simulink model "Assem4"  (R2018b)
(part 2 of 15)

  Revolute50 : sm_lib/Joints/Revolute Joint  SenseConstraintForce=off  SenseConstraintForceX=off  SenseConstraintForceY=off  SenseConstraintForceZ=off  SenseConstraintTorque=off  SenseConstraintTorqueX=off  SenseConstraintTorqueY=off  SenseConstraintTorqueZ=off  SenseTotalForce=off  SenseTotalForceX=off  SenseTotalForceY=off  SenseTotalForceZ=off  SenseTotalTorque=off  SenseTotalTorqueX=off  SenseTotalTorqueY=off  SenseTotalTorqueZ=off  CompositeWrenchDir=FollowerOnBase  CompositeWrenchFrame=BaseFrame  EquilibriumPosition=0  EquilibriumPositionUnits=rad  SpringStiffness=0  SpringStiffnessUnits=N*m/rad  DampingCoefficient=0  DampingCoefficientUnits=N*m/(rad/s)  TorqueActuationMode=NoTorque  MotionActuationMode=ComputedMotion  SensePosition=off  SenseVelocity=off  SenseAcceleration=off  SenseTorqueForce=off  PositionTargetSpecify=on  PositionTargetPriority=Low  PositionTargetValue=smiData.RevoluteJoint(51).Rz.Pos  PositionTargetValueUnits=deg  VelocityTargetSpecify=off  VelocityTargetPriority=High  VelocityTargetValue=0  VelocityTargetValueUnits=deg/s
  Revolute51 : sm_lib/Joints/Revolute Joint  SenseConstraintForce=off  SenseConstraintForceX=off  SenseConstraintForceY=off  SenseConstraintForceZ=off  SenseConstraintTorque=off  SenseConstraintTorqueX=off  SenseConstraintTorqueY=off  SenseConstraintTorqueZ=off  SenseTotalForce=off  SenseTotalForceX=off  SenseTotalForceY=off  SenseTotalForceZ=off  SenseTotalTorque=off  SenseTotalTorqueX=off  SenseTotalTorqueY=off  SenseTotalTorqueZ=off  CompositeWrenchDir=FollowerOnBase  CompositeWrenchFrame=BaseFrame  EquilibriumPosition=0  EquilibriumPositionUnits=rad  SpringStiffness=0  SpringStiffnessUnits=N*m/rad  DampingCoefficient=0  DampingCoefficientUnits=N*m/(rad/s)  TorqueActuationMode=NoTorque  MotionActuationMode=ComputedMotion  SensePosition=off  SenseVelocity=off  SenseAcceleration=off  SenseTorqueForce=off  PositionTargetSpecify=on  PositionTargetPriority=Low  PositionTargetValue=smiData.RevoluteJoint(52).Rz.Pos  PositionTargetValueUnits=deg  VelocityTargetSpecify=off  VelocityTargetPriority=High  VelocityTargetValue=0  VelocityTargetValueUnits=deg/s
  Revolute52 : sm_lib/Joints/Revolute Joint  SenseConstraintForce=off  SenseConstraintForceX=off  SenseConstraintForceY=off  SenseConstraintForceZ=off  SenseConstraintTorque=off  SenseConstraintTorqueX=off  SenseConstraintTorqueY=off  SenseConstraintTorqueZ=off  SenseTotalForce=off  SenseTotalForceX=off  SenseTotalForceY=off  SenseTotalForceZ=off  SenseTotalTorque=off  SenseTotalTorqueX=off  SenseTotalTorqueY=off  SenseTotalTorqueZ=off  CompositeWrenchDir=FollowerOnBase  CompositeWrenchFrame=BaseFrame  EquilibriumPosition=0  EquilibriumPositionUnits=rad  SpringStiffness=0  SpringStiffnessUnits=N*m/rad  DampingCoefficient=0  DampingCoefficientUnits=N*m/(rad/s)  TorqueActuationMode=NoTorque  MotionActuationMode=ComputedMotion  SensePosition=off  SenseVelocity=off  SenseAcceleration=off  SenseTorqueForce=off  PositionTargetSpecify=on  PositionTargetPriority=Low  PositionTargetValue=smiData.RevoluteJoint(53).Rz.Pos  PositionTargetValueUnits=deg  VelocityTargetSpecify=off  VelocityTargetPriority=High  VelocityTargetValue=0  VelocityTargetValueUnits=deg/s
  Revolute53 : sm_lib/Joints/Revolute Joint  SenseConstraintForce=off  SenseConstraintForceX=off  SenseConstraintForceY=off  SenseConstraintForceZ=off  SenseConstraintTorque=off  SenseConstraintTorqueX=off  SenseConstraintTorqueY=off  SenseConstraintTorqueZ=off  SenseTotalForce=off  SenseTotalForceX=off  SenseTotalForceY=off  SenseTotalForceZ=off  SenseTotalTorque=off  SenseTotalTorqueX=off  SenseTotalTorqueY=off  SenseTotalTorqueZ=off  CompositeWrenchDir=FollowerOnBase  CompositeWrenchFrame=BaseFrame  EquilibriumPosition=0  EquilibriumPositionUnits=rad  SpringStiffness=0  SpringStiffnessUnits=N*m/rad  DampingCoefficient=0  DampingCoefficientUnits=N*m/(rad/s)  TorqueActuationMode=NoTorque  MotionActuationMode=ComputedMotion  SensePosition=off  SenseVelocity=off  SenseAcceleration=off  SenseTorqueForce=off  PositionTargetSpecify=on  PositionTargetPriority=Low  PositionTargetValue=smiData.RevoluteJoint(54).Rz.Pos  PositionTargetValueUnits=deg  VelocityTargetSpecify=off  VelocityTargetPriority=High  VelocityTargetValue=0  VelocityTargetValueUnits=deg/s
  Revolute54 : sm_lib/Joints/Revolute Joint  SenseConstraintForce=off  SenseConstraintForceX=off  SenseConstraintForceY=off  SenseConstraintForceZ=off  SenseConstraintTorque=off  SenseConstraintTorqueX=off  SenseConstraintTorqueY=off  SenseConstraintTorqueZ=off  SenseTotalForce=off  SenseTotalForceX=off  SenseTotalForceY=off  SenseTotalForceZ=off  SenseTotalTorque=off  SenseTotalTorqueX=off  SenseTotalTorqueY=off  SenseTotalTorqueZ=off  CompositeWrenchDir=FollowerOnBase  CompositeWrenchFrame=BaseFrame  EquilibriumPosition=0  EquilibriumPositionUnits=rad  SpringStiffness=0  SpringStiffnessUnits=N*m/rad  DampingCoefficient=0  DampingCoefficientUnits=N*m/(rad/s)  TorqueActuationMode=NoTorque  MotionActuationMode=ComputedMotion  SensePosition=off  SenseVelocity=off  SenseAcceleration=off  SenseTorqueForce=off  PositionTargetSpecify=on  PositionTargetPriority=Low  PositionTargetValue=smiData.RevoluteJoint(55).Rz.Pos  PositionTargetValueUnits=deg  VelocityTargetSpecify=off  VelocityTargetPriority=High  VelocityTargetValue=0  VelocityTargetValueUnits=deg/s
  Revolute55 : sm_lib/Joints/Revolute Joint  SenseConstraintForce=off  SenseConstraintForceX=off  SenseConstraintForceY=off  SenseConstraintForceZ=off  SenseConstraintTorque=off  SenseConstraintTorqueX=off  SenseConstraintTorqueY=off  SenseConstraintTorqueZ=off  SenseTotalForce=off  SenseTotalForceX=off  SenseTotalForceY=off  SenseTotalForceZ=off  SenseTotalTorque=off  SenseTotalTorqueX=off  SenseTotalTorqueY=off  SenseTotalTorqueZ=off  CompositeWrenchDir=FollowerOnBase  CompositeWrenchFrame=BaseFrame  EquilibriumPosition=0  EquilibriumPositionUnits=rad  SpringStiffness=0  SpringStiffnessUnits=N*m/rad  DampingCoefficient=0  DampingCoefficientUnits=N*m/(rad/s)  TorqueActuationMode=NoTorque  MotionActuationMode=ComputedMotion  SensePosition=off  SenseVelocity=off  SenseAcceleration=off  SenseTorqueForce=off  PositionTargetSpecify=on  PositionTargetPriority=Low  PositionTargetValue=smiData.RevoluteJoint(56).Rz.Pos  PositionTargetValueUnits=deg  VelocityTargetSpecify=off  VelocityTargetPriority=High  VelocityTargetValue=0  VelocityTargetValueUnits=deg/s
  Revolute56 : sm_lib/Joints/Revolute Joint  SenseConstraintForce=off  SenseConstraintForceX=off  SenseConstraintForceY=off  SenseConstraintForceZ=off  SenseConstraintTorque=off  SenseConstraintTorqueX=off  SenseConstraintTorqueY=off  SenseConstraintTorqueZ=off  SenseTotalForce=off  SenseTotalForceX=off  SenseTotalForceY=off  SenseTotalForceZ=off  SenseTotalTorque=off  SenseTotalTorqueX=off  SenseTotalTorqueY=off  SenseTotalTorqueZ=off  CompositeWrenchDir=FollowerOnBase  CompositeWrenchFrame=BaseFrame  EquilibriumPosition=0  EquilibriumPositionUnits=rad  SpringStiffness=0  SpringStiffnessUnits=N*m/rad  DampingCoefficient=0  DampingCoefficientUnits=N*m/(rad/s)  TorqueActuationMode=NoTorque  MotionActuationMode=ComputedMotion  SensePosition=off  SenseVelocity=off  SenseAcceleration=off  SenseTorqueForce=off  PositionTargetSpecify=on  PositionTargetPriority=Low  PositionTargetValue=smiData.RevoluteJoint(57).Rz.Pos  PositionTargetValueUnits=deg  VelocityTargetSpecify=off  VelocityTargetPriority=High  VelocityTargetValue=0  VelocityTargetValueUnits=deg/s
  Revolute57 : sm_lib/Joints/Revolute Joint  SenseConstraintForce=off  SenseConstraintForceX=off  SenseConstraintForceY=off  SenseConstraintForceZ=off  SenseConstraintTorque=off  SenseConstraintTorqueX=off  SenseConstraintTorqueY=off  SenseConstraintTorqueZ=off  SenseTotalForce=off  SenseTotalForceX=off  SenseTotalForceY=off  SenseTotalForceZ=off  SenseTotalTorque=off  SenseTotalTorqueX=off  SenseTotalTorqueY=off  SenseTotalTorqueZ=off  CompositeWrenchDir=FollowerOnBase  CompositeWrenchFrame=BaseFrame  EquilibriumPosition=0  EquilibriumPositionUnits=rad  SpringStiffness=0  SpringStiffnessUnits=N*m/rad  DampingCoefficient=0  DampingCoefficientUnits=N*m/(rad/s)  TorqueActuationMode=NoTorque  MotionActuationMode=ComputedMotion  SensePosition=off  SenseVelocity=off  SenseAcceleration=off  SenseTorqueForce=off  PositionTargetSpecify=on  PositionTargetPriority=Low  PositionTargetValue=smiData.RevoluteJoint(58).Rz.Pos  PositionTargetValueUnits=deg  VelocityTargetSpecify=off  VelocityTargetPriority=High  VelocityTargetValue=0  VelocityTargetValueUnits=deg/s
  Revolute58 : sm_lib/Joints/Revolute Joint  SenseConstraintForce=off  SenseConstraintForceX=off  SenseConstraintForceY=off  SenseConstraintForceZ=off  SenseConstraintTorque=off  SenseConstraintTorqueX=off  SenseConstraintTorqueY=off  SenseConstraintTorqueZ=off  SenseTotalForce=off  SenseTotalForceX=off  SenseTotalForceY=off  SenseTotalForceZ=off  SenseTotalTorque=off  SenseTotalTorqueX=off  SenseTotalTorqueY=off  SenseTotalTorqueZ=off  CompositeWrenchDir=FollowerOnBase  CompositeWrenchFrame=BaseFrame  EquilibriumPosition=0  EquilibriumPositionUnits=rad  SpringStiffness=0  SpringStiffnessUnits=N*m/rad  DampingCoefficient=0  DampingCoefficientUnits=N*m/(rad/s)  TorqueActuationMode=NoTorque  MotionActuationMode=ComputedMotion  SensePosition=off  SenseVelocity=off  SenseAcceleration=off  SenseTorqueForce=off  PositionTargetSpecify=on  PositionTargetPriority=Low  PositionTargetValue=smiData.RevoluteJoint(59).Rz.Pos  PositionTargetValueUnits=deg  VelocityTargetSpecify=off  VelocityTargetPriority=High  VelocityTargetValue=0  VelocityTargetValueUnits=deg/s
  Revolute59 : sm_lib/Joints/Revolute Joint  SenseConstraintForce=off  SenseConstraintForceX=off  SenseConstraintForceY=off  SenseConstraintForceZ=off  SenseConstraintTorque=off  SenseConstraintTorqueX=off  SenseConstraintTorqueY=off  SenseConstraintTorqueZ=off  SenseTotalForce=off  SenseTotalForceX=off  SenseTotalForceY=off  SenseTotalForceZ=off  SenseTotalTorque=off  SenseTotalTorqueX=off  SenseTotalTorqueY=off  SenseTotalTorqueZ=off  CompositeWrenchDir=FollowerOnBase  CompositeWrenchFrame=BaseFrame  EquilibriumPosition=0  EquilibriumPositionUnits=rad  SpringStiffness=0  SpringStiffnessUnits=N*m/rad  DampingCoefficient=0  DampingCoefficientUnits=N*m/(rad/s)  TorqueActuationMode=NoTorque  MotionActuationMode=ComputedMotion  SensePosition=off  SenseVelocity=off  SenseAcceleration=off  SenseTorqueForce=off  PositionTargetSpecify=on  PositionTargetPriority=Low  PositionTargetValue=smiData.RevoluteJoint(60).Rz.Pos  PositionTargetValueUnits=deg  VelocityTargetSpecify=off  VelocityTargetPriority=High  VelocityTargetValue=0  VelocityTargetValueUnits=deg/s
  Revolute6 : sm_lib/Joints/Revolute Joint  SenseConstraintForce=off  SenseConstraintForceX=off  SenseConstraintForceY=off  SenseConstraintForceZ=off  SenseConstraintTorque=off  SenseConstraintTorqueX=off  SenseConstraintTorqueY=off  SenseConstraintTorqueZ=off  SenseTotalForce=off  SenseTotalForceX=off  SenseTotalForceY=off  SenseTotalForceZ=off  SenseTotalTorque=off  SenseTotalTorqueX=off  SenseTotalTorqueY=off  SenseTotalTorqueZ=off  CompositeWrenchDir=FollowerOnBase  CompositeWrenchFrame=BaseFrame  EquilibriumPosition=0  EquilibriumPositionUnits=rad  SpringStiffness=0  SpringStiffnessUnits=N*m/rad  DampingCoefficient=0  DampingCoefficientUnits=N*m/(rad/s)  TorqueActuationMode=NoTorque  MotionActuationMode=ComputedMotion  SensePosition=off  SenseVelocity=off  SenseAcceleration=off  SenseTorqueForce=off  PositionTargetSpecify=on  PositionTargetPriority=Low  PositionTargetValue=smiData.RevoluteJoint(7).Rz.Pos  PositionTargetValueUnits=deg  VelocityTargetSpecify=off  VelocityTargetPriority=High  VelocityTargetValue=0  VelocityTargetValueUnits=deg/s
  Revolute60 : sm_lib/Joints/Revolute Joint  SenseConstraintForce=off  SenseConstraintForceX=off  SenseConstraintForceY=off  SenseConstraintForceZ=off  SenseConstraintTorque=off  SenseConstraintTorqueX=off  SenseConstraintTorqueY=off  SenseConstraintTorqueZ=off  SenseTotalForce=off  SenseTotalForceX=off  SenseTotalForceY=off  SenseTotalForceZ=off  SenseTotalTorque=off  SenseTotalTorqueX=off  SenseTotalTorqueY=off  SenseTotalTorqueZ=off  CompositeWrenchDir=FollowerOnBase  CompositeWrenchFrame=BaseFrame  EquilibriumPosition=0  EquilibriumPositionUnits=rad  SpringStiffness=0  SpringStiffnessUnits=N*m/rad  DampingCoefficient=0  DampingCoefficientUnits=N*m/(rad/s)  TorqueActuationMode=NoTorque  MotionActuationMode=ComputedMotion  SensePosition=off  SenseVelocity=off  SenseAcceleration=off  SenseTorqueForce=off  PositionTargetSpecify=on  PositionTargetPriority=Low  PositionTargetValue=smiData.RevoluteJoint(61).Rz.Pos  PositionTargetValueUnits=deg  VelocityTargetSpecify=off  VelocityTargetPriority=High  VelocityTargetValue=0  VelocityTargetValueUnits=deg/s
  Revolute61 : sm_lib/Joints/Revolute Joint  SenseConstraintForce=off  SenseConstraintForceX=off  SenseConstraintForceY=off  SenseConstraintForceZ=off  SenseConstraintTorque=off  SenseConstraintTorqueX=off  SenseConstraintTorqueY=off  SenseConstraintTorqueZ=off  SenseTotalForce=off  SenseTotalForceX=off  SenseTotalForceY=off  SenseTotalForceZ=off  SenseTotalTorque=off  SenseTotalTorqueX=off  SenseTotalTorqueY=off  SenseTotalTorqueZ=off  CompositeWrenchDir=FollowerOnBase  CompositeWrenchFrame=BaseFrame  EquilibriumPosition=0  EquilibriumPositionUnits=rad  SpringStiffness=0  SpringStiffnessUnits=N*m/rad  DampingCoefficient=0  DampingCoefficientUnits=N*m/(rad/s)  TorqueActuationMode=NoTorque  MotionActuationMode=ComputedMotion  SensePosition=off  SenseVelocity=off  SenseAcceleration=off  SenseTorqueForce=off  PositionTargetSpecify=on  PositionTargetPriority=Low  PositionTargetValue=smiData.RevoluteJoint(62).Rz.Pos  PositionTargetValueUnits=deg  VelocityTargetSpecify=off  VelocityTargetPriority=High  VelocityTargetValue=0  VelocityTargetValueUnits=deg/s
  Revolute62 : sm_lib/Joints/Revolute Joint  SenseConstraintForce=off  SenseConstraintForceX=off  SenseConstraintForceY=off  SenseConstraintForceZ=off  SenseConstraintTorque=off  SenseConstraintTorqueX=off  SenseConstraintTorqueY=off  SenseConstraintTorqueZ=off  SenseTotalForce=off  SenseTotalForceX=off  SenseTotalForceY=off  SenseTotalForceZ=off  SenseTotalTorque=off  SenseTotalTorqueX=off  SenseTotalTorqueY=off  SenseTotalTorqueZ=off  CompositeWrenchDir=FollowerOnBase  CompositeWrenchFrame=BaseFrame  EquilibriumPosition=0  EquilibriumPositionUnits=rad  SpringStiffness=0  SpringStiffnessUnits=N*m/rad  DampingCoefficient=0  DampingCoefficientUnits=N*m/(rad/s)  TorqueActuationMode=NoTorque  MotionActuationMode=ComputedMotion  SensePosition=off  SenseVelocity=off  SenseAcceleration=off  SenseTorqueForce=off  PositionTargetSpecify=on  PositionTargetPriority=Low  PositionTargetValue=smiData.RevoluteJoint(63).Rz.Pos  PositionTargetValueUnits=deg  VelocityTargetSpecify=off  VelocityTargetPriority=High  VelocityTargetValue=0  VelocityTargetValueUnits=deg/s
  Revolute63 : sm_lib/Joints/Revolute Joint  SenseConstraintForce=off  SenseConstraintForceX=off  SenseConstraintForceY=off  SenseConstraintForceZ=off  SenseConstraintTorque=off  SenseConstraintTorqueX=off  SenseConstraintTorqueY=off  SenseConstraintTorqueZ=off  SenseTotalForce=off  SenseTotalForceX=off  SenseTotalForceY=off  SenseTotalForceZ=off  SenseTotalTorque=off  SenseTotalTorqueX=off  SenseTotalTorqueY=off  SenseTotalTorqueZ=off  CompositeWrenchDir=FollowerOnBase  CompositeWrenchFrame=BaseFrame  EquilibriumPosition=0  EquilibriumPositionUnits=rad  SpringStiffness=0  SpringStiffnessUnits=N*m/rad  DampingCoefficient=0  DampingCoefficientUnits=N*m/(rad/s)  TorqueActuationMode=NoTorque  MotionActuationMode=ComputedMotion  SensePosition=off  SenseVelocity=off  SenseAcceleration=off  SenseTorqueForce=off  PositionTargetSpecify=on  PositionTargetPriority=Low  PositionTargetValue=smiData.RevoluteJoint(64).Rz.Pos  PositionTargetValueUnits=deg  VelocityTargetSpecify=off  VelocityTargetPriority=High  VelocityTargetValue=0  VelocityTargetValueUnits=deg/s
  Revolute64 : sm_lib/Joints/Revolute Joint  SenseConstraintForce=off  SenseConstraintForceX=off  SenseConstraintForceY=off  SenseConstraintForceZ=off  SenseConstraintTorque=off  SenseConstraintTorqueX=off  SenseConstraintTorqueY=off  SenseConstraintTorqueZ=off  SenseTotalForce=off  SenseTotalForceX=off  SenseTotalForceY=off  SenseTotalForceZ=off  SenseTotalTorque=off  SenseTotalTorqueX=off  SenseTotalTorqueY=off  SenseTotalTorqueZ=off  CompositeWrenchDir=FollowerOnBase  CompositeWrenchFrame=BaseFrame  EquilibriumPosition=0  EquilibriumPositionUnits=rad  SpringStiffness=0  SpringStiffnessUnits=N*m/rad  DampingCoefficient=0  DampingCoefficientUnits=N*m/(rad/s)  TorqueActuationMode=NoTorque  MotionActuationMode=ComputedMotion  SensePosition=off  SenseVelocity=off  SenseAcceleration=off  SenseTorqueForce=off  PositionTargetSpecify=on  PositionTargetPriority=Low  PositionTargetValue=smiData.RevoluteJoint(65).Rz.Pos  PositionTargetValueUnits=deg  VelocityTargetSpecify=off  VelocityTargetPriority=High  VelocityTargetValue=0  VelocityTargetValueUnits=deg/s
  Revolute65 : sm_lib/Joints/Revolute Joint  SenseConstraintForce=off  SenseConstraintForceX=off  SenseConstraintForceY=off  SenseConstraintForceZ=off  SenseConstraintTorque=off  SenseConstraintTorqueX=off  SenseConstraintTorqueY=off  SenseConstraintTorqueZ=off  SenseTotalForce=off  SenseTotalForceX=off  SenseTotalForceY=off  SenseTotalForceZ=off  SenseTotalTorque=off  SenseTotalTorqueX=off  SenseTotalTorqueY=off  SenseTotalTorqueZ=off  CompositeWrenchDir=FollowerOnBase  CompositeWrenchFrame=BaseFrame  EquilibriumPosition=0  EquilibriumPositionUnits=rad  SpringStiffness=0  SpringStiffnessUnits=N*m/rad  DampingCoefficient=0  DampingCoefficientUnits=N*m/(rad/s)  TorqueActuationMode=NoTorque  MotionActuationMode=ComputedMotion  SensePosition=off  SenseVelocity=off  SenseAcceleration=off  SenseTorqueForce=off  PositionTargetSpecify=on  PositionTargetPriority=Low  PositionTargetValue=smiData.RevoluteJoint(66).Rz.Pos  PositionTargetValueUnits=deg  VelocityTargetSpecify=off  VelocityTargetPriority=High  VelocityTargetValue=0  VelocityTargetValueUnits=deg/s
  Revolute66 : sm_lib/Joints/Revolute Joint  SenseConstraintForce=off  SenseConstraintForceX=off  SenseConstraintForceY=off  SenseConstraintForceZ=off  SenseConstraintTorque=off  SenseConstraintTorqueX=off  SenseConstraintTorqueY=off  SenseConstraintTorqueZ=off  SenseTotalForce=off  SenseTotalForceX=off  SenseTotalForceY=off  SenseTotalForceZ=off  SenseTotalTorque=off  SenseTotalTorqueX=off  SenseTotalTorqueY=off  SenseTotalTorqueZ=off  CompositeWrenchDir=FollowerOnBase  CompositeWrenchFrame=BaseFrame  EquilibriumPosition=0  EquilibriumPositionUnits=rad  SpringStiffness=0  SpringStiffnessUnits=N*m/rad  DampingCoefficient=0  DampingCoefficientUnits=N*m/(rad/s)  TorqueActuationMode=NoTorque  MotionActuationMode=ComputedMotion  SensePosition=off  SenseVelocity=off  SenseAcceleration=off  SenseTorqueForce=off  PositionTargetSpecify=on  PositionTargetPriority=Low  PositionTargetValue=smiData.RevoluteJoint(67).Rz.Pos  PositionTargetValueUnits=deg  VelocityTargetSpecify=off  VelocityTargetPriority=High  VelocityTargetValue=0  VelocityTargetValueUnits=deg/s
  Revolute67 : sm_lib/Joints/Revolute Joint  SenseConstraintForce=off  SenseConstraintForceX=off  SenseConstraintForceY=off  SenseConstraintForceZ=off  SenseConstraintTorque=off  SenseConstraintTorqueX=off  SenseConstraintTorqueY=off  SenseConstraintTorqueZ=off  SenseTotalForce=off  SenseTotalForceX=off  SenseTotalForceY=off  SenseTotalForceZ=off  SenseTotalTorque=off  SenseTotalTorqueX=off  SenseTotalTorqueY=off  SenseTotalTorqueZ=off  CompositeWrenchDir=FollowerOnBase  CompositeWrenchFrame=BaseFrame  EquilibriumPosition=0  EquilibriumPositionUnits=rad  SpringStiffness=0  SpringStiffnessUnits=N*m/rad  DampingCoefficient=0  DampingCoefficientUnits=N*m/(rad/s)  TorqueActuationMode=NoTorque  MotionActuationMode=ComputedMotion  SensePosition=off  SenseVelocity=off  SenseAcceleration=off  SenseTorqueForce=off  PositionTargetSpecify=on  PositionTargetPriority=Low  PositionTargetValue=smiData.RevoluteJoint(68).Rz.Pos  PositionTargetValueUnits=deg  VelocityTargetSpecify=off  VelocityTargetPriority=High  VelocityTargetValue=0  VelocityTargetValueUnits=deg/s
  Revolute68 : sm_lib/Joints/Revolute Joint  SenseConstraintForce=off  SenseConstraintForceX=off  SenseConstraintForceY=off  SenseConstraintForceZ=off  SenseConstraintTorque=off  SenseConstraintTorqueX=off  SenseConstraintTorqueY=off  SenseConstraintTorqueZ=off  SenseTotalForce=off  SenseTotalForceX=off  SenseTotalForceY=off  SenseTotalForceZ=off  SenseTotalTorque=off  SenseTotalTorqueX=off  SenseTotalTorqueY=off  SenseTotalTorqueZ=off  CompositeWrenchDir=FollowerOnBase  CompositeWrenchFrame=BaseFrame  EquilibriumPosition=0  EquilibriumPositionUnits=rad  SpringStiffness=0  SpringStiffnessUnits=N*m/rad  DampingCoefficient=0  DampingCoefficientUnits=N*m/(rad/s)  TorqueActuationMode=NoTorque  MotionActuationMode=ComputedMotion  SensePosition=off  SenseVelocity=off  SenseAcceleration=off  SenseTorqueForce=off  PositionTargetSpecify=on  PositionTargetPriority=Low  PositionTargetValue=smiData.RevoluteJoint(69).Rz.Pos  PositionTargetValueUnits=deg  VelocityTargetSpecify=off  VelocityTargetPriority=High  VelocityTargetValue=0  VelocityTargetValueUnits=deg/s
  Revolute69 : sm_lib/Joints/Revolute Joint  SenseConstraintForce=off  SenseConstraintForceX=off  SenseConstraintForceY=off  SenseConstraintForceZ=off  SenseConstraintTorque=off  SenseConstraintTorqueX=off  SenseConstraintTorqueY=off  SenseConstraintTorqueZ=off  SenseTotalForce=off  SenseTotalForceX=off  SenseTotalForceY=off  SenseTotalForceZ=off  SenseTotalTorque=off  SenseTotalTorqueX=off  SenseTotalTorqueY=off  SenseTotalTorqueZ=off  CompositeWrenchDir=FollowerOnBase  CompositeWrenchFrame=BaseFrame  EquilibriumPosition=0  EquilibriumPositionUnits=rad  SpringStiffness=0  SpringStiffnessUnits=N*m/rad  DampingCoefficient=0  DampingCoefficientUnits=N*m/(rad/s)  TorqueActuationMode=NoTorque  MotionActuationMode=ComputedMotion  SensePosition=off  SenseVelocity=off  SenseAcceleration=off  SenseTorqueForce=off  PositionTargetSpecify=on  PositionTargetPriority=Low  PositionTargetValue=smiData.RevoluteJoint(70).Rz.Pos  PositionTargetValueUnits=deg  VelocityTargetSpecify=off  VelocityTargetPriority=High  VelocityTargetValue=0  VelocityTargetValueUnits=deg/s
  Revolute7 : sm_lib/Joints/Revolute Joint  SenseConstraintForce=off  SenseConstraintForceX=off  SenseConstraintForceY=off  SenseConstraintForceZ=off  SenseConstraintTorque=off  SenseConstraintTorqueX=off  SenseConstraintTorqueY=off  SenseConstraintTorqueZ=off  SenseTotalForce=off  SenseTotalForceX=off  SenseTotalForceY=off  SenseTotalForceZ=off  SenseTotalTorque=off  SenseTotalTorqueX=off  SenseTotalTorqueY=off  SenseTotalTorqueZ=off  CompositeWrenchDir=FollowerOnBase  CompositeWrenchFrame=BaseFrame  EquilibriumPosition=0  EquilibriumPositionUnits=rad  SpringStiffness=0  SpringStiffnessUnits=N*m/rad  DampingCoefficient=0  DampingCoefficientUnits=N*m/(rad/s)  TorqueActuationMode=NoTorque  MotionActuationMode=ComputedMotion  SensePosition=off  SenseVelocity=off  SenseAcceleration=off  SenseTorqueForce=off  PositionTargetSpecify=on  PositionTargetPriority=Low  PositionTargetValue=smiData.RevoluteJoint(8).Rz.Pos  PositionTargetValueUnits=deg  VelocityTargetSpecify=off  VelocityTargetPriority=High  VelocityTargetValue=0  VelocityTargetValueUnits=deg/s
  Revolute8 : sm_lib/Joints/Revolute Joint  SenseConstraintForce=off  SenseConstraintForceX=off  SenseConstraintForceY=off  SenseConstraintForceZ=off  SenseConstraintTorque=off  SenseConstraintTorqueX=off  SenseConstraintTorqueY=off  SenseConstraintTorqueZ=off  SenseTotalForce=off  SenseTotalForceX=off  SenseTotalForceY=off  SenseTotalForceZ=off  SenseTotalTorque=off  SenseTotalTorqueX=off  SenseTotalTorqueY=off  SenseTotalTorqueZ=off  CompositeWrenchDir=FollowerOnBase  CompositeWrenchFrame=BaseFrame  EquilibriumPosition=0  EquilibriumPositionUnits=rad  SpringStiffness=0  SpringStiffnessUnits=N*m/rad  DampingCoefficient=0  DampingCoefficientUnits=N*m/(rad/s)  TorqueActuationMode=NoTorque  MotionActuationMode=ComputedMotion  SensePosition=off  SenseVelocity=off  SenseAcceleration=off  SenseTorqueForce=off  PositionTargetSpecify=on  PositionTargetPriority=Low  PositionTargetValue=smiData.RevoluteJoint(9).Rz.Pos  PositionTargetValueUnits=deg  VelocityTargetSpecify=off  VelocityTargetPriority=High  VelocityTargetValue=0  VelocityTargetValueUnits=deg/s
  Revolute9 : sm_lib/Joints/Revolute Joint  SenseConstraintForce=off  SenseConstraintForceX=off  SenseConstraintForceY=off  SenseConstraintForceZ=off  SenseConstraintTorque=off  SenseConstraintTorqueX=off  SenseConstraintTorqueY=off  SenseConstraintTorqueZ=off  SenseTotalForce=off  SenseTotalForceX=off  SenseTotalForceY=off  SenseTotalForceZ=off  SenseTotalTorque=off  SenseTotalTorqueX=off  SenseTotalTorqueY=off  SenseTotalTorqueZ=off  CompositeWrenchDir=FollowerOnBase  CompositeWrenchFrame=BaseFrame  EquilibriumPosition=0  EquilibriumPositionUnits=rad  SpringStiffness=0  SpringStiffnessUnits=N*m/rad  DampingCoefficient=0  DampingCoefficientUnits=N*m/(rad/s)  TorqueActuationMode=NoTorque  MotionActuationMode=ComputedMotion  SensePosition=off  SenseVelocity=off  SenseAcceleration=off  SenseTorqueForce=off  PositionTargetSpecify=on  PositionTargetPriority=Low  PositionTargetValue=smiData.RevoluteJoint(10).Rz.Pos  PositionTargetValueUnits=deg  VelocityTargetSpecify=off  VelocityTargetPriority=High  VelocityTargetValue=0  VelocityTargetValueUnits=deg/s
  Solver Configuration : nesl_utility/Solver Configuration  PhysicalDomain=network_engine_domain  SubClassName=solver  LeftPortType=input  RightPortType=generic  Tones=[]  Harmonics=[]  SimulateNoise=off  Profile=off  UseLocalSampling=off  EnableSwitchedLinearOptims=on  FrequencyDomain=off  UseCCode=off  RelTol=0.001  AbsTol=1e-06  MinStep=1e-09  ToWorkspace=off  RevertToSquareIcSolve=off  NumHomotopyIterations=100  PhasorMode=off  PhasorModeNumHarmonics=1  DoDC=off  ResidualTolerance=1e-09  UseLocalSolver=off  LocalSolverChoice=NE_BACKWARD_EULER_ADVANCER  LocalSolverSampleTime=0.001  DoFixedCost=off  MaxNonlinIter=3  MaxModeIter=2  LinearAlgebra=auto  EquationFormulation=NE_TIME_EF  DelaysMemoryBudget=1024  AutomaticFiltering=on  FilteringTimeConstant=0.001  PartitionStorageMethod=AS_NEEDED  PartitionMemoryBudget=1024
  Transform : sm_lib/Frames and Transforms/Rigid Transform  TranslationMethod=Cartesian  TranslationStandardOffset=0  TranslationLengthUnit=mm  TranslationStandardAxis=+Z  TranslationCartesianOffset=smiData.RigidTransform(377).translation  TranslationROffset=0  TranslationROffsetUnits=m  TranslationZOffset=0  TranslationZOffsetUnits=m  TranslationThetaOffset=0  TranslationThetaOffsetUnits=deg  RotationMethod=ArbitraryAxis  RotationAngleUnits=rad  RotationStandardAxis=+Z  RotationAngle=smiData.RigidTransform(377).angle  RotationArbitraryAxis=smiData.RigidTransform(377).axis  FollAlignAxisA=+X  BaseAlignAxisA=+Y  FollAlignAxisB=+Y  BaseAlignAxisB=+Z  RotationSequenceAxes=FollowerAxes  RotationSequence=XYX  RotationSequenceAngles=[0 0 0]  RotationSequenceAnglesUnits=deg  RotationMatrix=[1 0 0; 0 1 0; 0 0 1]
  World : sm_lib/Frames and Transforms/World Frame
  hex_flange_machine_screw_am_10_RIGID : Subsystem
  hex_flange_machine_screw_am_11_RIGID : Subsystem
  hex_flange_machine_screw_am_12_RIGID : Subsystem
  hex_flange_machine_screw_am_13_RIGID : Subsystem
  hex_flange_machine_screw_am_18_RIGID : Subsystem
  hex_flange_machine_screw_am_19_RIGID : Subsystem
  hex_flange_machine_screw_am_20_RIGID : Subsystem
  hex_flange_machine_screw_am_21_RIGID : Subsystem
  hex_flange_machine_screw_am_22_RIGID : Subsystem
  hex_flange_machine_screw_am_23_RIGID : Subsystem
  hex_flange_machine_screw_am_24_RIGID : Subsystem
  hex_flange_machine_screw_am_25_RIGID : Subsystem
  hex_flange_machine_screw_am_26_RIGID : Subsystem
  hex_flange_machine_screw_am_27_RIGID : Subsystem
  hex_flange_machine_screw_am_28_RIGID : Subsystem
  hex_flange_machine_screw_am_29_RIGID : Subsystem
  hex_flange_machine_screw_am_2_RIGID : Subsystem
  hex_flange_machine_screw_am_3_RIGID : Subsystem
  hex_flange_machine_screw_am_4_RIGID : Subsystem
  hex_flange_machine_screw_am_5_RIGID : Subsystem
  hex_flange_machine_screw_am_6_RIGID : Subsystem
  hex_flange_machine_screw_am_7_RIGID : Subsystem
  hex_flange_machine_screw_am_8_RIGID : Subsystem
  hex_flange_machine_screw_am_9_RIGID : Subsystem
  hex_flange_nut_am_10_RIGID : Subsystem
  hex_flange_nut_am_11_RIGID : Subsystem
  hex_flange_nut_am_12_RIGID : Subsystem
  hex_flange_nut_am_13_RIGID : Subsystem
  hex_flange_nut_am_14_RIGID : Subsystem
  hex_flange_nut_am_16_RIGID : Subsystem
  hex_flange_nut_am_17_RIGID : Subsystem
  hex_flange_nut_am_18_RIGID : Subsystem
  hex_flange_nut_am_1_RIGID : Subsystem
  hex_flange_nut_am_20_RIGID : Subsystem
  hex_flange_nut_am_21_RIGID : Subsystem
  hex_flange_nut_am_23_RIGID : Subsystem
  hex_flange_nut_am_24_RIGID : Subsystem
  hex_flange_nut_am_25_RIGID : Subsystem
  hex_flange_nut_am_26_RIGID : Subsystem
  hex_flange_nut_am_27_RIGID : Subsystem
  hex_flange_nut_am_28_RIGID : Subsystem
  hex_flange_nut_am_29_RIGID : Subsystem
  hex_flange_nut_am_2_RIGID : Subsystem
  hex_flange_nut_am_3_RIGID : Subsystem
  hex_flange_nut_am_6_RIGID : Subsystem
  hex_flange_nut_am_7_RIGID : Subsystem
  hex_flange_nut_am_8_RIGID : Subsystem
  hex_flange_nut_am_9_RIGID : Subsystem
  instrument_ball_bearing_68_am_12_RIGID : Subsystem
  instrument_ball_bearing_68_am_13_RIGID : Subsystem
  instrument_ball_bearing_68_am_15_RIGID : Subsystem
  instrument_ball_bearing_68_am_16_RIGID : Subsystem
  instrument_ball_bearing_68_am_17_RIGID : Subsystem
  instrument_ball_bearing_68_am_18_RIGID : Subsystem
  instrument_ball_bearing_68_am_1_RIGID : Subsystem
  instrument_ball_bearing_68_am_20_RIGID : Subsystem
  instrument_ball_bearing_68_am_21_RIGID : Subsystem
  instrument_ball_bearing_68_am_22_RIGID : Subsystem
  instrument_ball_bearing_68_am_23_RIGID : Subsystem
  instrument_ball_bearing_68_am_24_RIGID : Subsystem
  instrument_ball_bearing_68_am_25_RIGID : Subsystem
  instrument_ball_bearing_68_am_4_RIGID : Subsystem
  instrument_ball_bearing_68_am_6_RIGID : Subsystem
  kafa3_1_RIGID : Subsystem
  mafsal_10_RIGID : Subsystem
  mafsal_11_RIGID : Subsystem
  mafsal_13_RIGID : Subsystem
  mafsal_14_RIGID : Subsystem
  mafsal_15_RIGID : Subsystem
  mafsal_1_RIGID : Subsystem
  mafsal_2_RIGID : Subsystem
  mafsal_3_RIGID : Subsystem
  mafsal_4_RIGID : Subsystem
  mafsal_5_RIGID : Subsystem
  mafsal_8_RIGID : Subsystem
  mafsal_9_RIGID : Subsystem
  para6_1_RIGID : Subsystem
  connections:
  Transform/LConn1 -- Mechanism Configuration/RConn1 -- Solver Configuration/RConn1 -- World/RConn1
  Part10_1_RIGID/RConn10 -- Prismatic/LConn1
  Revolute3/RConn1 -- hex_flange_machine_screw_am_5_RIGID/LConn1
  Revolute29/RConn1 -- instrument_ball_bearing_68_am_22_RIGID/LConn1
  Revolute30/LConn1 -- para6_1_RIGID/RConn2
  Revolute30/RConn1 -- instrument_ball_bearing_68_am_23_RIGID/LConn1
  Revolute31/LConn1 -- para6_1_RIGID/RConn1
  Revolute31/RConn1 -- instrument_ball_bearing_68_am_24_RIGID/LConn1
  Revolute32/LConn1 -- para6_1_RIGID/RConn6
  Revolute32/RConn1 -- instrument_ball_bearing_68_am_25_RIGID/LConn1
  Planar10/LConn1 -- mafsal_9_RIGID/RConn2
  Planar10/RConn1 -- para6_1_RIGID/LConn7
  Kopya_Moteur_1_RIGID/RConn5 -- Planar11/LConn1
  Cylindrical/LConn1 -- kafa3_1_RIGID/RConn15
  Planar11/RConn1 -- hex_flange_nut_am_16_RIGID/LConn2
  Kopya_Moteur_1_RIGID/RConn4 -- Planar12/LConn1
  Planar12/RConn1 -- hex_flange_nut_am_17_RIGID/LConn2
  Kopya_Moteur_1_RIGID/RConn1 -- Planar13/LConn1
  Planar13/RConn1 -- hex_flange_nut_am_18_RIGID/LConn2
  Kopya_Moteur_1_RIGID/RConn2 -- Planar14/LConn1
  Planar14/RConn1 -- hex_flange_nut_am_20_RIGID/LConn2
  Kopya_Moteur_2_RIGID/RConn5 -- Planar15/LConn1
  Planar15/RConn1 -- hex_flange_nut_am_21_RIGID/LConn1
  Kopya_Moteur_2_RIGID/RConn4 -- Planar16/LConn1
  Cylindrical/RConn1 -- Part10_1_RIGID/LConn1
  Planar16/RConn1 -- hex_flange_nut_am_23_RIGID/LConn2
  Kopya_Moteur_2_RIGID/RConn3 -- Planar17/LConn1
  Planar17/RConn1 -- hex_flange_nut_am_24_RIGID/LConn2
  Kopya_Moteur_2_RIGID/RConn2 -- Revolute33/LConn1
  Revolute33/RConn1 -- hex_flange_nut_am_25_RIGID/LConn1
  Kopya_Moteur_3_RIGID/RConn5 -- Planar18/LConn1
  Planar18/RConn1 -- hex_flange_nut_am_26_RIGID/LConn1
  Kopya_Moteur_3_RIGID/RConn4 -- Planar19/LConn1
  Planar19/RConn1 -- hex_flange_nut_am_27_RIGID/LConn2
  Kopya_Moteur_3_RIGID/RConn3 -- Planar20/LConn1
  Part10_2_RIGID/RConn10 -- Prismatic1/LConn1
  Planar20/RConn1 -- hex_flange_nut_am_28_RIGID/LConn2
  Kopya_Moteur_3_RIGID/RConn2 -- Planar21/LConn1
  Planar21/RConn1 -- hex_flange_nut_am_29_RIGID/LConn2
  Part10_3_RIGID/RConn8 -- Revolute34/LConn1
  Revolute34/RConn1 -- hex_flange_machine_screw_am_10_RIGID/LConn1
  Cylindrical7/LConn1 -- hex_flange_machine_screw_am_10_RIGID/RConn1
  Cylindrical7/RConn1 -- hex_flange_nut_am_14_RIGID/LConn2
  Part10_3_RIGID/RConn6 -- Revolute35/LConn1
  Revolute35/RConn1 -- hex_flange_machine_screw_am_11_RIGID/LConn1
  Cylindrical8/LConn1 -- hex_flange_machine_screw_am_11_RIGID/RConn1
  Kopya_Moteur_2_RIGID/LConn1 -- Prismatic1/RConn1
  Cylindrical8/RConn1 -- hex_flange_nut_am_3_RIGID/LConn1
  Part10_3_RIGID/RConn4 -- Revolute36/LConn1
  Revolute36/RConn1 -- hex_flange_machine_screw_am_12_RIGID/LConn1
  Cylindrical9/LConn1 -- hex_flange_machine_screw_am_12_RIGID/RConn1
  Cylindrical9/RConn1 -- hex_flange_nut_am_2_RIGID/LConn1
  Part10_3_RIGID/RConn2 -- Revolute37/LConn1
  Revolute37/RConn1 -- hex_flange_machine_screw_am_13_RIGID/LConn1
  Cylindrical10/LConn1 -- hex_flange_machine_screw_am_13_RIGID/RConn1
  Cylindrical10/RConn1 -- hex_flange_nut_am_1_RIGID/LConn1
  Part10_2_RIGID/RConn6 -- Revolute38/LConn1
  Part10_2_RIGID/RConn8 -- Revolute4/LConn1
  Revolute38/RConn1 -- hex_flange_machine_screw_am_18_RIGID/LConn1
  Cylindrical11/LConn1 -- hex_flange_machine_screw_am_18_RIGID/RConn1
  Cylindrical11/RConn1 -- hex_flange_nut_am_21_RIGID/LConn2
  Part10_2_RIGID/RConn3 -- Revolute39/LConn1
  Revolute39/RConn1 -- hex_flange_machine_screw_am_19_RIGID/LConn1
  Part10_2_RIGID/RConn1 -- Revolute40/LConn1
  Revolute40/RConn1 -- hex_flange_machine_screw_am_20_RIGID/LConn1
  Cylindrical12/LConn1 -- hex_flange_machine_screw_am_20_RIGID/RConn1
  Cylindrical12/RConn1 -- hex_flange_nut_am_24_RIGID/LConn1
  Part10_2_RIGID/RConn2 -- Revolute41/LConn1
  Revolute4/RConn1 -- hex_flange_machine_screw_am_6_RIGID/LConn1
  Revolute41/RConn1 -- hex_flange_machine_screw_am_21_RIGID/LConn1
  Cylindrical13/LConn1 -- hex_flange_machine_screw_am_21_RIGID/RConn1
  Cylindrical13/RConn1 -- hex_flange_nut_am_23_RIGID/LConn1
  Part10_3_RIGID/RConn5 -- Revolute42/LConn1
  Revolute42/RConn1 -- hex_flange_machine_screw_am_22_RIGID/LConn1
  Cylindrical14/LConn1 -- hex_flange_machine_screw_am_22_RIGID/RConn1
  Cylindrical14/RConn1 -- hex_flange_nut_am_17_RIGID/LConn1
  Part10_3_RIGID/RConn3 -- Revolute43/LConn1
  Revolute43/RConn1 -- hex_flange_machine_screw_am_23_RIGID/LConn1
  Cylindrical15/LConn1 -- hex_flange_machine_screw_am_23_RIGID/RConn1
  Part10_2_RIGID/RConn7 -- Revolute5/LConn1
  Cylindrical15/RConn1 -- hex_flange_nut_am_16_RIGID/LConn1
  Part10_3_RIGID/RConn1 -- Revolute44/LConn1
  Revolute44/RConn1 -- hex_flange_machine_screw_am_24_RIGID/LConn1
  Cylindrical16/LConn1 -- hex_flange_machine_screw_am_24_RIGID/RConn1
  Cylindrical16/RConn1 -- hex_flange_nut_am_18_RIGID/LConn1
  Part10_3_RIGID/RConn7 -- Revolute45/LConn1
  Revolute45/RConn1 -- hex_flange_machine_screw_am_25_RIGID/LConn1
  Cylindrical17/LConn1 -- hex_flange_machine_screw_am_25_RIGID/RConn1
  Cylindrical17/RConn1 -- hex_flange_nut_am_20_RIGID/LConn1
  Part10_1_RIGID/RConn6 -- Revolute46/LConn1
  Revolute5/RConn1 -- hex_flange_machine_screw_am_7_RIGID/LConn1
  Revolute46/RConn1 -- hex_flange_machine_screw_am_26_RIGID/LConn1
  Cylindrical18/LConn1 -- hex_flange_machine_screw_am_26_RIGID/RConn1
  Cylindrical18/RConn1 -- hex_flange_nut_am_26_RIGID/LConn2
  Part10_1_RIGID/RConn3 -- Revolute47/LConn1
  Revolute47/RConn1 -- hex_flange_machine_screw_am_27_RIGID/LConn1
  Cylindrical19/LConn1 -- hex_flange_machine_screw_am_27_RIGID/RConn1
  Cylindrical19/RConn1 -- hex_flange_nut_am_28_RIGID/LConn1
  Part10_1_RIGID/RConn2 -- Revolute48/LConn1
  Revolute48/RConn1 -- hex_flange_machine_screw_am_28_RIGID/LConn1
  Cylindrical20/LConn1 -- hex_flange_machine_screw_am_28_RIGID/RConn1
  Part10_2_RIGID/RConn5 -- Revolute6/LConn1
  Cylindrical20/RConn1 -- hex_flange_nut_am_29_RIGID/LConn1
  Part10_1_RIGID/RConn1 -- Revolute49/LConn1
  Revolute49/RConn1 -- hex_flange_machine_screw_am_29_RIGID/LConn1
  Cylindrical21/LConn1 -- hex_flange_machine_screw_am_29_RIGID/RConn1
  Cylindrical21/RConn1 -- hex_flange_nut_am_27_RIGID/LConn1
  Cylindrical22/LConn1 -- Para2_4_RIGID/RConn2
  Cylindrical22/RConn1 -- instrument_ball_bearing_68_am_12_RIGID/LConn1
  Cylindrical23/LConn1 -- Para2_4_RIGID/RConn1
  Cylindrical23/RConn1 -- instrument_ball_bearing_68_am_13_RIGID/LConn1
  Cylindrical24/LConn1 -- Para2_1_RIGID/RConn2
  Kopya_Moteur_3_RIGID/LConn1 -- Prismatic/RConn1
  Revolute6/RConn1 -- hex_flange_machine_screw_am_8_RIGID/LConn1
  Cylindrical24/RConn1 -- instrument_ball_bearing_68_am_15_RIGID/LConn1
  Cylindrical25/LConn1 -- Para2_1_RIGID/RConn1
  Cylindrical25/RConn1 -- instrument_ball_bearing_68_am_16_RIGID/LConn1
  Cylindrical26/LConn1 -- Para2_2_RIGID/RConn3
  Cylindrical26/RConn1 -- instrument_ball_bearing_68_am_17_RIGID/LConn1
  Cylindrical27/LConn1 -- Para2_2_RIGID/RConn2
  Cylindrical27/RConn1 -- instrument_ball_bearing_68_am_18_RIGID/LConn1
  Revolute50/LConn1 -- kafa3_1_RIGID/RConn14
  Revolute50/RConn1 -- hex_flange_nut_am_10_RIGID/LConn1
  Revolute51/LConn1 -- kafa3_1_RIGID/RConn12
  Part10_2_RIGID/RConn4 -- Revolute7/LConn1
  Revolute51/RConn1 -- hex_flange_nut_am_11_RIGID/LConn1
  Cylindrical28/LConn1 -- hex_flange_machine_screw_am_6_RIGID/RConn1
  Cylindrical28/RConn1 -- hex_flange_nut_am_12_RIGID/LConn2
  Planar22/LConn1 -- kafa3_1_RIGID/RConn9
  Planar22/RConn1 -- hex_flange_nut_am_12_RIGID/LConn1
  Cylindrical29/LConn1 -- hex_flange_machine_screw_am_7_RIGID/RConn1
  Cylindrical29/RConn1 -- hex_flange_nut_am_13_RIGID/LConn2
  Planar23/LConn1 -- kafa3_1_RIGID/RConn8
  Planar23/RConn1 -- hex_flange_nut_am_13_RIGID/LConn1
  Planar24/LConn1 -- kafa3_1_RIGID/RConn6
  Revolute7/RConn1 -- hex_flange_machine_screw_am_9_RIGID/LConn1
  Planar24/RConn1 -- hex_flange_nut_am_14_RIGID/LConn1
  Para4_4_RIGID/RConn1 -- Revolute52/LConn1
  Para1_10_RIGID/LConn1 -- Revolute52/RConn1
  Para4_5_RIGID/RConn1 -- Revolute53/LConn1
  Para1_11_RIGID/LConn2 -- Revolute53/RConn1
  Para4_6_RIGID/RConn1 -- Revolute54/LConn1
  Para1_12_RIGID/LConn1 -- Revolute54/RConn1
  Para1_1_RIGID/RConn1 -- Revolute55/LConn1
  Para4_4_RIGID/LConn1 -- Revolute55/RConn1
  Revolute56/LConn1 -- mafsal_2_RIGID/RConn2
  Cylindrical1/LConn1 -- kafa3_1_RIGID/RConn13
  Para1_1_RIGID/LConn1 -- Revolute56/RConn1
  Para1_2_RIGID/RConn1 -- Revolute57/LConn1
  Para4_3_RIGID/LConn1 -- Revolute57/RConn1
  Revolute58/LConn1 -- mafsal_1_RIGID/RConn3
  Para1_2_RIGID/LConn1 -- Revolute58/RConn1
  Para1_3_RIGID/RConn1 -- Revolute59/LConn1
  Para4_5_RIGID/LConn1 -- Revolute59/RConn1
  Para1_3_RIGID/RConn2 -- Planar25/LConn1
  Planar25/RConn1 -- mafsal_3_RIGID/LConn2
  Para1_4_RIGID/RConn1 -- Revolute60/LConn1
  Cylindrical1/RConn1 -- Part10_2_RIGID/LConn1
  Para4_1_RIGID/LConn1 -- Revolute60/RConn1
  Revolute61/LConn1 -- mafsal_8_RIGID/RConn2
  Para1_4_RIGID/LConn1 -- Revolute61/RConn1
  Para1_5_RIGID/RConn1 -- Revolute62/LConn1
  Para4_2_RIGID/LConn1 -- Revolute62/RConn1
  Revolute63/LConn1 -- mafsal_5_RIGID/RConn2
  Para1_5_RIGID/LConn1 -- Revolute63/RConn1
  Para1_6_RIGID/RConn1 -- Revolute64/LConn1
  Para4_6_RIGID/LConn1 -- Revolute64/RConn1
  Revolute65/LConn1 -- mafsal_4_RIGID/RConn1
  Part10_3_RIGID/RConn10 -- Prismatic2/LConn1
  Para1_6_RIGID/LConn1 -- Revolute65/RConn1
  Para4_1_RIGID/RConn1 -- Revolute66/LConn1
  Para1_7_RIGID/LConn1 -- Revolute66/RConn1
  Para4_2_RIGID/RConn1 -- Revolute67/LConn1
  Para1_8_RIGID/LConn1 -- Revolute67/RConn1
  Para4_3_RIGID/RConn1 -- Revolute68/LConn1
  Para1_9_RIGID/LConn1 -- Revolute68/RConn1
  Revolute69/LConn1 -- mafsal_9_RIGID/RConn1
  Para1_9_RIGID/LConn2 -- Revolute69/RConn1
  Planar26/LConn1 -- mafsal_1_RIGID/RConn1
  Kopya_Moteur_1_RIGID/LConn1 -- Prismatic2/RConn1
  Para2_1_RIGID/LConn2 -- Planar26/RConn1
  Planar27/LConn1 -- mafsal_2_RIGID/RConn1
  Para2_1_RIGID/LConn4 -- Planar27/RConn1
  Planar28/LConn1 -- mafsal_3_RIGID/RConn2
  Para2_2_RIGID/LConn3 -- Planar28/RConn1
  Para2_2_RIGID/RConn1 -- Planar29/LConn1
  Planar29/RConn1 -- mafsal_4_RIGID/LConn1
  Planar30/LConn1 -- mafsal_5_RIGID/RConn1
  Para2_4_RIGID/LConn4 -- Planar30/RConn1
  Planar31/LConn1 -- mafsal_8_RIGID/RConn1
  Cylindrical2/LConn1 -- kafa3_1_RIGID/RConn7
  Para2_4_RIGID/LConn1 -- Planar31/RConn1
  Cylindrical30/LConn1 -- instrument_ball_bearing_68_am_16_RIGID/RConn1
  Cylindrical30/RConn1 -- Part2_1_RIGID/LConn1
  Part2_1_RIGID/RConn3 -- Planar32/LConn1
  Para2_1_RIGID/LConn3 -- Planar32/RConn1
  Cylindrical31/LConn1 -- Part2_1_RIGID/RConn2
  Cylindrical31/RConn1 -- mafsal_1_RIGID/LConn1
  Cylindrical32/LConn1 -- Part2_1_RIGID/RConn1
  Cylindrical32/RConn1 -- mafsal_2_RIGID/LConn1
  Cylindrical33/LConn1 -- instrument_ball_bearing_68_am_13_RIGID/RConn1
  Cylindrical2/RConn1 -- Part10_3_RIGID/LConn1
  Cylindrical33/RConn1 -- Part2_2_RIGID/LConn1
  Part2_2_RIGID/RConn3 -- Planar33/LConn1
  Para2_4_RIGID/LConn2 -- Planar33/RConn1
  Cylindrical34/LConn1 -- Part2_2_RIGID/RConn2
  Cylindrical34/RConn1 -- mafsal_5_RIGID/LConn1
  Cylindrical35/LConn1 -- Part2_2_RIGID/RConn1
  Cylindrical35/RConn1 -- mafsal_8_RIGID/LConn1
  Cylindrical36/LConn1 -- instrument_ball_bearing_68_am_18_RIGID/RConn1
  Cylindrical36/RConn1 -- Part2_3_RIGID/LConn1
  Part2_3_RIGID/RConn3 -- Planar34/LConn1
  Cylindrical3/LConn1 -- Part10_3_RIGID/RConn9
  Para2_2_RIGID/LConn2 -- Planar34/RConn1
  Cylindrical37/LConn1 -- Part2_3_RIGID/RConn2
  Cylindrical37/RConn1 -- mafsal_3_RIGID/LConn1
  Cylindrical38/LConn1 -- Part2_3_RIGID/RConn1
  Cylindrical38/RConn1 -- mafsal_4_RIGID/LConn2
  Cylindrical39/LConn1 -- Part2_4_RIGID/RConn3
  Cylindrical39/RConn1 -- mafsal_13_RIGID/LConn1
  Cylindrical40/LConn1 -- Part2_4_RIGID/RConn2
  Cylindrical40/RConn1 -- mafsal_15_RIGID/LConn1
  Part2_4_RIGID/RConn1 -- Planar35/LConn1
  Part10_1_RIGID/RConn9 -- Revolute/LConn1
  Cylindrical3/RConn1 -- instrument_ball_bearing_68_am_4_RIGID/LConn1
  Planar35/RConn1 -- para6_1_RIGID/LConn5
  Cylindrical41/LConn1 -- instrument_ball_bearing_68_am_20_RIGID/RConn1
  Cylindrical41/RConn1 -- Part2_4_RIGID/LConn1
  Cylindrical42/LConn1 -- Part2_5_RIGID/RConn3
  Cylindrical42/RConn1 -- mafsal_10_RIGID/LConn1
  Part2_5_RIGID/RConn2 -- Planar36/LConn1
  Planar36/RConn1 -- para6_1_RIGID/LConn8
  Cylindrical43/LConn1 -- instrument_ball_bearing_68_am_25_RIGID/RConn1
  Cylindrical43/RConn1 -- Part2_5_RIGID/LConn1
  Cylindrical44/LConn1 -- Part2_5_RIGID/RConn1
  Cylindrical4/LConn1 -- Part12_1_RIGID/RConn1
  Cylindrical44/RConn1 -- mafsal_9_RIGID/LConn1
  Cylindrical45/LConn1 -- Part2_6_RIGID/RConn3
  Cylindrical45/RConn1 -- mafsal_11_RIGID/LConn1
  Cylindrical46/LConn1 -- Part2_6_RIGID/RConn1
  Cylindrical46/RConn1 -- mafsal_14_RIGID/LConn1
  Part2_6_RIGID/RConn2 -- Planar37/LConn1
  Planar37/RConn1 -- para6_1_RIGID/LConn3
  Cylindrical47/LConn1 -- instrument_ball_bearing_68_am_23_RIGID/RConn1
  Cylindrical47/RConn1 -- Part2_6_RIGID/LConn1
  Cylindrical48/LConn1 -- Part10_1_RIGID/RConn8
  Cylindrical4/RConn1 -- Para1_3_RIGID/LConn1
  Cylindrical48/RConn1 -- Part9_1_RIGID/LConn3
  Kopya_Moteur_3_RIGID/RConn1 -- Planar38/LConn1
  Part9_1_RIGID/LConn2 -- Planar38/RConn1
  Para2_2_RIGID/LConn1 -- Part9_1_RIGID/LConn1
  Cylindrical49/LConn1 -- Part9_1_RIGID/RConn1
  Cylindrical49/RConn1 -- instrument_ball_bearing_68_am_6_RIGID/LConn1
  Cylindrical50/LConn1 -- Part10_2_RIGID/RConn9
  Cylindrical50/RConn1 -- Part9_2_RIGID/LConn3
  Kopya_Moteur_2_RIGID/RConn1 -- Planar39/LConn1
  Part9_2_RIGID/LConn2 -- Planar39/RConn1
  Revolute8/LConn1 -- mafsal_3_RIGID/RConn1
  Para2_4_RIGID/LConn3 -- Part9_2_RIGID/LConn1
  Cylindrical51/LConn1 -- Part9_2_RIGID/RConn1
  Cylindrical51/RConn1 -- instrument_ball_bearing_68_am_1_RIGID/LConn1
  Kopya_Moteur_1_RIGID/RConn3 -- Planar40/LConn1
  Part9_3_RIGID/LConn1 -- Planar40/RConn1
  Para2_1_RIGID/LConn1 -- Part9_3_RIGID/LConn3
  Cylindrical52/LConn1 -- instrument_ball_bearing_68_am_4_RIGID/RConn1
  Cylindrical52/RConn1 -- Part9_3_RIGID/LConn2
  Transform/RConn1 -- kafa3_1_RIGID/LConn1
  Part12_1_RIGID/LConn1 -- Revolute8/RConn1
  Revolute9/LConn1 -- mafsal_2_RIGID/RConn3
  Part12_2_RIGID/LConn1 -- Revolute9/RConn1
  Revolute10/LConn1 -- mafsal_4_RIGID/RConn2
  Part12_3_RIGID/LConn1 -- Revolute10/RConn1
  Revolute11/LConn1 -- mafsal_1_RIGID/RConn2
  Revolute/RConn1 -- hex_flange_machine_screw_am_2_RIGID/LConn1
  Part12_4_RIGID/LConn1 -- Revolute11/RConn1
  Revolute12/LConn1 -- mafsal_5_RIGID/RConn3
  Part12_5_RIGID/LConn1 -- Revolute12/RConn1
  Revolute13/LConn1 -- mafsal_8_RIGID/RConn3
  Part12_6_RIGID/LConn1 -- Revolute13/RConn1
  Revolute14/LConn1 -- mafsal_13_RIGID/RConn3
  Part12_7_RIGID/LConn1 -- Revolute14/RConn1
  Revolute15/LConn1 -- mafsal_15_RIGID/RConn3
  Part12_8_RIGID/LConn1 -- Revolute15/RConn1
  Revolute16/LConn1 -- mafsal_14_RIGID/RConn2
  Part10_1_RIGID/RConn4 -- Revolute1/LConn1
  Part12_9_RIGID/LConn1 -- Revolute16/RConn1
  Planar/LConn1 -- kafa3_1_RIGID/RConn5
  Planar/RConn1 -- hex_flange_nut_am_1_RIGID/LConn2
  Planar1/LConn1 -- kafa3_1_RIGID/RConn4
  Planar1/RConn1 -- hex_flange_nut_am_2_RIGID/LConn2
  Planar2/LConn1 -- kafa3_1_RIGID/RConn3
  Planar2/RConn1 -- hex_flange_nut_am_3_RIGID/LConn2
  Cylindrical5/LConn1 -- hex_flange_machine_screw_am_2_RIGID/RConn1
  Cylindrical5/RConn1 -- hex_flange_nut_am_6_RIGID/LConn2
  Planar3/LConn1 -- kafa3_1_RIGID/RConn11
  Revolute1/RConn1 -- hex_flange_machine_screw_am_3_RIGID/LConn1
  Planar3/RConn1 -- hex_flange_nut_am_6_RIGID/LConn1
  Cylindrical6/LConn1 -- hex_flange_machine_screw_am_3_RIGID/RConn1
  Cylindrical6/RConn1 -- hex_flange_nut_am_7_RIGID/LConn2
  Planar4/LConn1 -- kafa3_1_RIGID/RConn10
  Planar4/RConn1 -- hex_flange_nut_am_7_RIGID/LConn1
  Revolute17/LConn1 -- kafa3_1_RIGID/RConn2
  Revolute17/RConn1 -- hex_flange_nut_am_8_RIGID/LConn1
  Revolute18/LConn1 -- kafa3_1_RIGID/RConn1
  Revolute18/RConn1 -- hex_flange_nut_am_9_RIGID/LConn1
  Revolute19/LConn1 -- mafsal_11_RIGID/RConn3
  Part10_1_RIGID/RConn7 -- Revolute2/LConn1
  Part12_10_RIGID/LConn1 -- Revolute19/RConn1
  Revolute20/LConn1 -- mafsal_10_RIGID/RConn3
  Part12_11_RIGID/LConn1 -- Revolute20/RConn1
  Revolute21/LConn1 -- mafsal_9_RIGID/RConn3
  Part12_12_RIGID/LConn1 -- Revolute21/RConn1
  Planar5/LConn1 -- mafsal_10_RIGID/RConn2
  Planar5/RConn1 -- para6_1_RIGID/LConn9
  Revolute22/LConn1 -- mafsal_10_RIGID/RConn1
  Para1_10_RIGID/LConn2 -- Revolute22/RConn1
  Planar6/LConn1 -- mafsal_11_RIGID/RConn2
  Revolute2/RConn1 -- hex_flange_machine_screw_am_4_RIGID/LConn1
  Planar6/RConn1 -- para6_1_RIGID/LConn1
  Revolute23/LConn1 -- mafsal_11_RIGID/RConn1
  Para1_12_RIGID/LConn2 -- Revolute23/RConn1
  Planar7/LConn1 -- mafsal_13_RIGID/RConn1
  Planar7/RConn1 -- para6_1_RIGID/LConn4
  Revolute24/LConn1 -- mafsal_13_RIGID/RConn2
  Para1_7_RIGID/LConn2 -- Revolute24/RConn1
  Planar8/LConn1 -- mafsal_14_RIGID/RConn1
  Planar8/RConn1 -- para6_1_RIGID/LConn6
  Revolute25/LConn1 -- mafsal_14_RIGID/RConn3
  Part10_1_RIGID/RConn5 -- Revolute3/LConn1
  Para1_11_RIGID/LConn1 -- Revolute25/RConn1
  Planar9/LConn1 -- mafsal_15_RIGID/RConn2
  Planar9/RConn1 -- para6_1_RIGID/LConn2
  Revolute26/LConn1 -- mafsal_15_RIGID/RConn1
  Para1_8_RIGID/LConn2 -- Revolute26/RConn1
  Revolute27/LConn1 -- para6_1_RIGID/RConn5
  Revolute27/RConn1 -- instrument_ball_bearing_68_am_20_RIGID/LConn1
  Revolute28/LConn1 -- para6_1_RIGID/RConn4
  Revolute28/RConn1 -- instrument_ball_bearing_68_am_21_RIGID/LConn1
  Revolute29/LConn1 -- para6_1_RIGID/RConn3
